simulink model "Task1simu"  (R2020b)
settings: Solver=VariableStepAuto  StartTime=0.0  StopTime=10  RelTol=1e-3
values from neighbouring files (symbols this model uses):
  A = [0,1,0,0;0,0,-m*g/M,0;0,0,0,1;0,0,(M+m)*g/(M*l),0]    [Task1.m]    (also in Task2.m = [-a*m1, a, 0)
  AGC = A-G*c    [Task1.m]
  b = [0;1/M;0;-1/(M*l)]    [Task1.m]    (also in Task2.m = 14.28)
  c = [1,0,0,0]    [Task1.m]    (also in Task2.m = 1)
  G = K2'    [Task1.m]
  K = place(A,b,P1)    [Task1.m]    (also in Task2.m = inv(P)*V)
  KH = K-c    [Task1.m]
  KH1 = K3(1,1:4)    [Task1.m]
  KH2 = -K3(1,5)    [Task1.m]
settings Model: Creator=CLINT  LastModifiedBy=CLINT

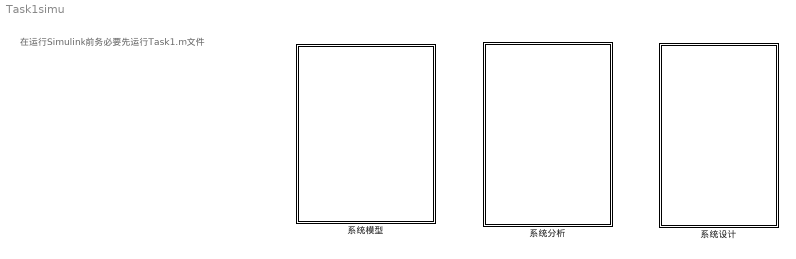
== system Task1simu ==
  note: 在运行Simulink前务必要先运行Task1.m文件
  系统分析 : Subsystem
  系统模型 : Subsystem
  系统设计 : Subsystem

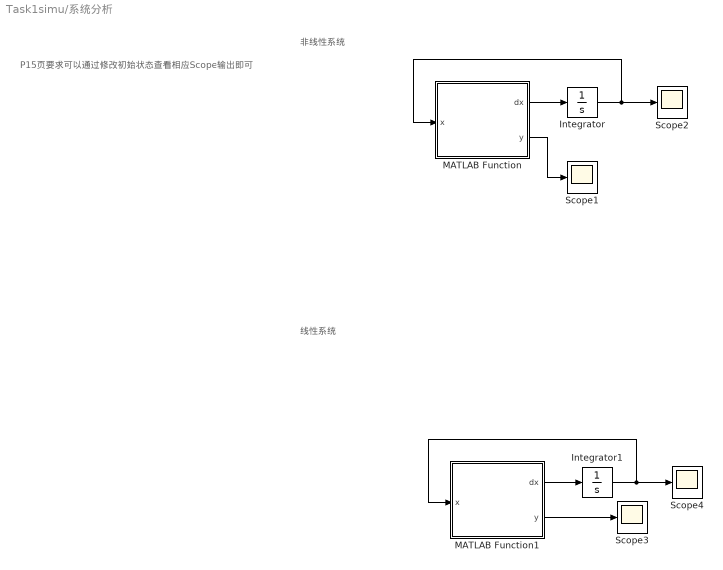
== system Task1simu/系统分析 ==
  note: P15页要求可以通过修改初始状态查看相应Scope输出即可
  note: 非线性系统
  note: 线性系统
  Integrator : Integrator  InitialCondition=[0;0;0.1;0]
  Integrator1 : Integrator  InitialCondition=[0;0;0.1;0]
  MATLAB Function : MATLAB Function  TreatAsAtomicUnit=on
  MATLAB Function1 : MATLAB Function  TreatAsAtomicUnit=on
  Scope{1..4} (4 alike) : Scope
  wires:
  MATLAB Function1/2(y) -> Scope3/1
  Integrator1/1 -> Scope4/1, MATLAB Function1/1(x)
  MATLAB Function/2(y) -> Scope1/1
  MATLAB Function/1(dx) -> Integrator/1
  Integrator/1 -> Scope2/1, MATLAB Function/1(x)
  MATLAB Function1/1(dx) -> Integrator1/1

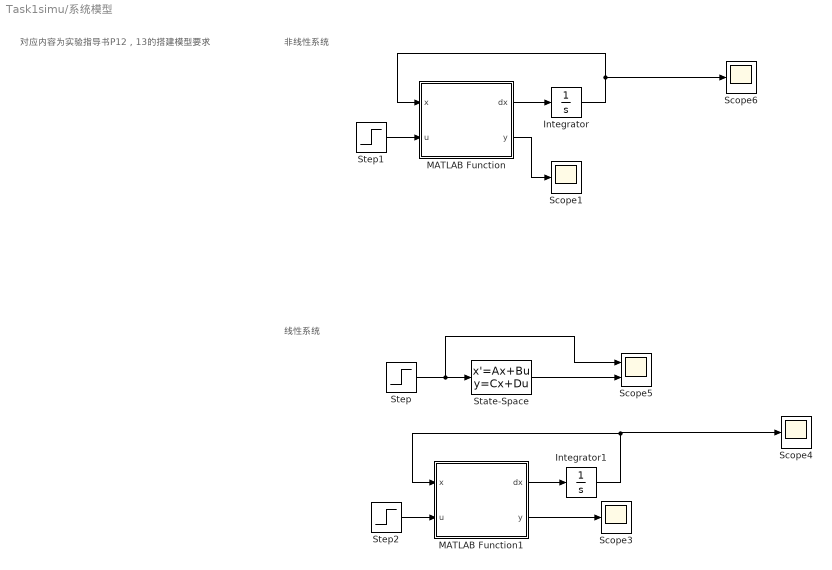
== system Task1simu/系统模型 ==
  note: 非线性系统
  note: 线性系统
  note: 对应内容为实验指导书P12，13的搭建模型要求
  Integrator : Integrator  InitialCondition=[0;0;0;0]
  Integrator1 : Integrator  InitialCondition=[0.1;0;0.1;0]
  MATLAB Function : MATLAB Function  TreatAsAtomicUnit=on
  MATLAB Function1 : MATLAB Function  TreatAsAtomicUnit=on
  Scope{1,3..4,6} (4 alike) : Scope
  Scope5 : Scope  NumInputPorts=2
  State-Space : StateSpace  A=A  B=b  C=c  D=0  InitialCondition=[0;0;0;0]
  Step : Step  SampleTime=0
  Step1 : Step  SampleTime=0
  Step2 : Step  SampleTime=0
  wires:
  MATLAB Function/1(dx) -> Integrator/1
  Step/1 -> Scope5/1, State-Space/1
  MATLAB Function1/1(dx) -> Integrator1/1
  MATLAB Function/2(y) -> Scope1/1
  Integrator1/1 -> Scope4/1, MATLAB Function1/1(x)
  MATLAB Function1/2(y) -> Scope3/1
  Step2/1 -> MATLAB Function1/2(u)
  State-Space/1 -> Scope5/2
  Integrator/1 -> Scope6/1, MATLAB Function/1(x)
  Step1/1 -> MATLAB Function/2(u)

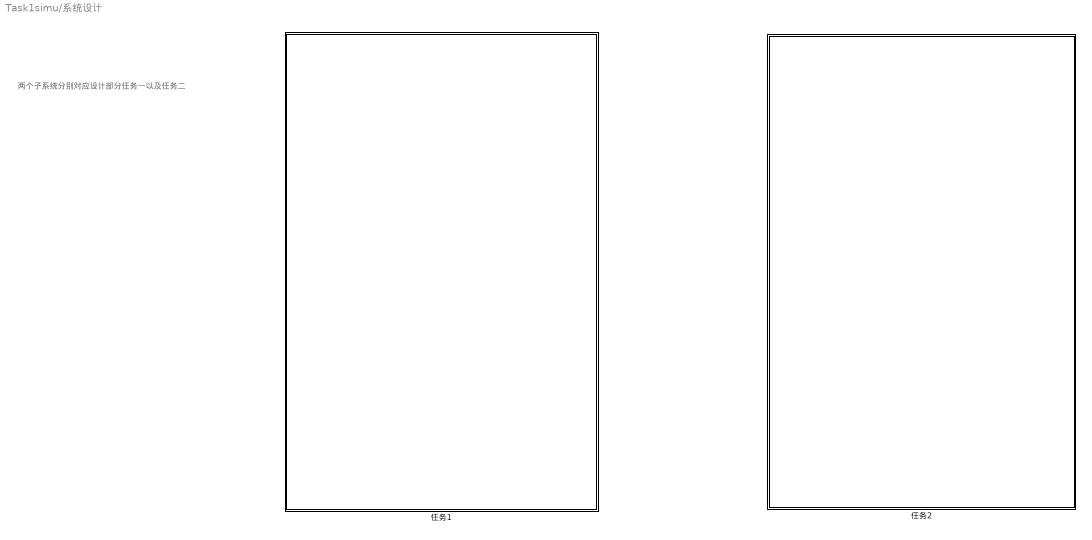
== system Task1simu/系统设计 ==
  note: 两个子系统分别对应设计部分任务一以及任务二
  任务1 : Subsystem
  任务2 : Subsystem

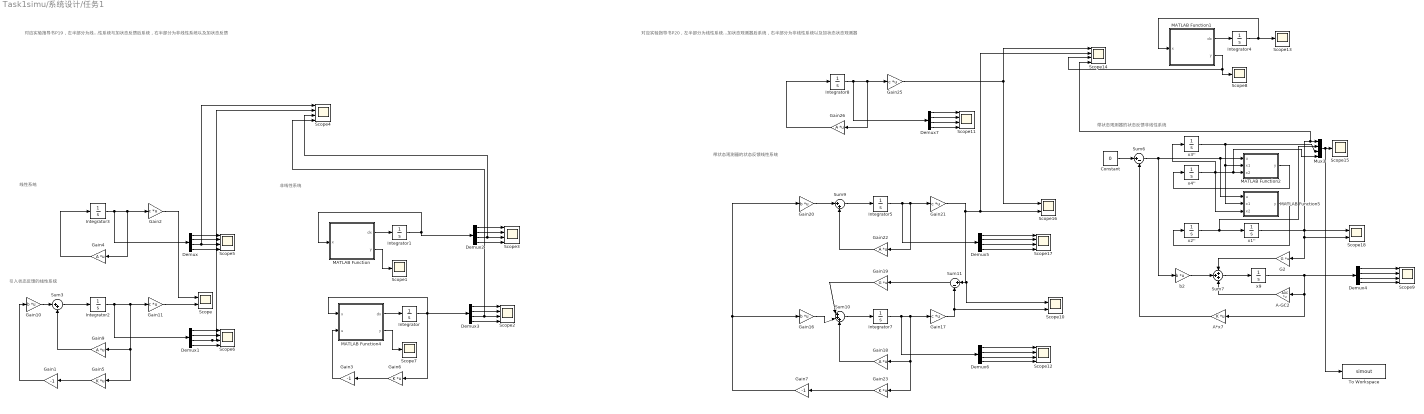
== system Task1simu/系统设计/任务1 ==
  note: 线性系统
  note: 引入状态反馈的线性系统
  note: 非线性系统
  note: 带状态观测器的状态反馈线性系统
  note: 带状态观测器的状态反馈非线性系统
  note: 对应实验指导书P19，左半部分为线性系统与加状态反馈后系统，右半部分为非线性系统以及加状态反馈
  note: 对应实验指导书P20，左半部分为线性系统与加状态观测器后系统，右半部分为非线性系统以及加状态状态观测器
  A*x7 : Gain  Gain=K  Multiplication=Matrix(K*u)
  A-GC2 : Gain  Gain=AGC  Multiplication=Matrix(K*u)
  Constant : Constant  Value=0
  Demux{,1..7} (8 alike) : Demux
  G2 : Gain  Gain=G  Multiplication=Matrix(K*u)
  Gain1 : Gain  Gain=-1
  Gain10 : Gain  Gain=b  Multiplication=Matrix(K*u)
  Gain{2,11,17,21,25} (5 alike) : Gain  Gain=c  Multiplication=Matrix(K*u)
  Gain16 : Gain  Gain=b  Multiplication=Matrix(K*u)
  Gain{4,9,18,22,26} (5 alike) : Gain  Gain=A  Multiplication=Matrix(K*u)
  Gain19 : Gain  Gain=G  Multiplication=Matrix(K*u)
  Gain20 : Gain  Gain=b  Multiplication=Matrix(K*u)
  Gain23 : Gain  Gain=K  Multiplication=Matrix(K*u)
  Gain3 : Gain  Gain=-1
  Gain5 : Gain  Gain=K  Multiplication=Matrix(K*u)
  Gain6 : Gain  Gain=K  Multiplication=Matrix(K*u)
  Gain7 : Gain  Gain=-1
  Integrator{,1..5,8} (7 alike) : Integrator  InitialCondition=[0;0;0.1;0]
  Integrator7 : Integrator  InitialCondition=[0;0.1;0;0.1]
  MATLAB Function : MATLAB Function  TreatAsAtomicUnit=on
  MATLAB Function1 : MATLAB Function  TreatAsAtomicUnit=on
  MATLAB Function2 : MATLAB Function  TreatAsAtomicUnit=on
  MATLAB Function4 : MATLAB Function  TreatAsAtomicUnit=on
  MATLAB Function5 : MATLAB Function  TreatAsAtomicUnit=on
  Mux3 : Mux
  Scope{,10,16,18} (4 alike) : Scope  NumInputPorts=2
  Scope{1,7..8,13,15} (5 alike) : Scope
  Scope{2..6,9,11..12,14,17} (10 alike) : Scope  NumInputPorts=4
  Sum10 : Sum  Inputs=|+++
  Sum11 : Sum  Inputs=|+-
  Sum3 : Sum  Inputs=|++
  Sum6 : Sum  Inputs=|+-
  Sum7 : Sum  Inputs=+++
  Sum9 : Sum  Inputs=|++
  To Workspace : ToWorkspace  VariableName=simout  SaveFormat=Timeseries  SampleTime=-1
  b2 : Gain  Gain=b  Multiplication=Matrix(K*u)
  x1'' : Integrator  InitialCondition=0.1
  x2'' : Integrator  InitialCondition=0.1
  x3'' : Integrator
  "x4'' " : Integrator
  x9 : Integrator  InitialCondition=0.1
  wires:
  Gain4/1 -> Integrator3/1
  Gain11/1 -> Scope/2
  Demux/1 -> Scope5/1
  Integrator2/1 -> Demux1/1, Gain11/1, Gain9/1, Gain5/1
  Integrator/1 -> MATLAB Function4/1(x), Demux3/1, Gain6/1
  Integrator3/1 -> Demux/1, Gain4/1, Gain2/1
  Demux/2 -> Scope5/2
  MATLAB Function/1(dx) -> Integrator1/1
  Demux2/2 -> Scope3/2
  Demux1/4 -> Scope6/4
  Integrator1/1 -> MATLAB Function/1(x), Demux2/1
  MATLAB Function4/2(y) -> Scope7/1
  Demux/3 -> Scope4/1, Scope5/3
  Gain2/1 -> Scope/1
  MATLAB Function/2(y) -> Scope1/1
  Gain5/1 -> Gain1/1
  Sum3/1 -> Integrator2/1
  Gain10/1 -> Sum3/1
  Gain9/1 -> Sum3/2
  Gain1/1 -> Gain10/1
  Demux1/3 -> Scope4/2, Scope6/3
  Demux3/3 -> Scope4/4, Scope2/3
  Demux2/1 -> Scope3/1
  Demux/4 -> Scope5/4
  Gain3/1 -> MATLAB Function4/2(u)
  Demux3/2 -> Scope2/2
  Demux2/3 -> Scope4/3, Scope3/3
  Demux3/4 -> Scope2/4
  Demux2/4 -> Scope3/4
  Demux1/1 -> Scope6/1
  Demux1/2 -> Scope6/2
  Demux3/1 -> Scope2/1
  MATLAB Function4/1(dx) -> Integrator/1
  Gain6/1 -> Gain3/1
  Demux6/2 -> Scope12/2
  Demux4/1 -> Scope9/1
  Gain26/1 -> Integrator8/1
  Gain20/1 -> Sum9/1
  Demux6/3 -> Scope12/3
  x1''/1 -> Scope18/2, G2/1, Scope18/1, Scope14/4, Mux3/1
  Demux4/2 -> Scope9/2
  Demux5/3 -> Scope17/3
  Demux5/1 -> Scope17/1
  Gain16/1 -> Sum10/2
  Demux7/4 -> Scope11/4
  MATLAB Function5/1(y) -> x2''/1
  Integrator7/1 -> Demux6/1, Gain23/1, Gain18/1, Gain17/1
  Demux6/4 -> Scope12/4
  Gain23/1 -> Gain7/1
  Demux7/3 -> Scope11/3
  MATLAB Function2/1(y) -> "x4'' "/1
  Mux3/1 -> To Workspace/1, Scope15/1
  Sum7/1 -> x9/1
  Demux4/3 -> Scope9/3
  Sum9/1 -> Integrator5/1
  Sum11/1 -> Gain19/1
  A*x7/1 -> Sum6/2
  Demux7/2 -> Scope11/2
  x3''/1 -> Mux3/3, MATLAB Function5/2(x1), MATLAB Function2/2(x1)
  "x4'' "/1 -> x3''/1, Mux3/4, MATLAB Function2/3(x2), MATLAB Function5/3(x2)
  Demux4/4 -> Scope9/4
  G2/1 -> Sum7/1
  Demux6/1 -> Scope12/1
  Gain22/1 -> Sum9/2
  b2/1 -> Sum7/2
  Sum10/1 -> Integrator7/1
  Gain19/1 -> Sum10/1
  Integrator5/1 -> Demux5/1, Gain22/1, Gain21/1
  Gain17/1 -> Sum11/2, Scope10/2
  Gain18/1 -> Sum10/3
  x2''/1 -> Mux3/2, x1''/1
  Gain7/1 -> Gain16/1, Gain20/1
  Constant/1 -> Sum6/1
  Gain21/1 -> Scope14/2, Scope16/2, Scope10/1, Sum11/1
  Integrator8/1 -> Demux7/1, Gain26/1, Gain25/1
  Demux7/1 -> Scope11/1
  Integrator4/1 -> Scope13/1, MATLAB Function1/1(x)
  x9/1 -> Demux4/1, A*x7/1, A-GC2/1
  Demux5/2 -> Scope17/2
  Sum6/1 -> MATLAB Function5/1(u), MATLAB Function2/1(u), b2/1
  Gain25/1 -> Scope16/1, Scope14/1
  Demux5/4 -> Scope17/4
  A-GC2/1 -> Sum7/3
  MATLAB Function1/1(dx) -> Integrator4/1
  MATLAB Function1/2(y) -> Scope14/3, Scope8/1

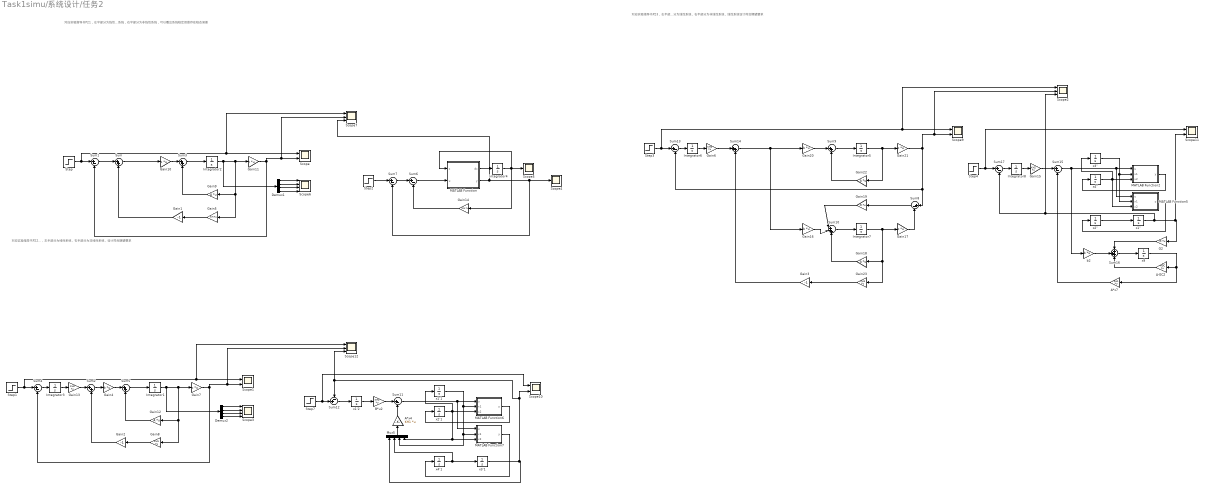
== system Task1simu/系统设计/任务2 ==
  note: 对应实验指导书P21，左半部分为线性系统，右半部分为非线性系统，可以看出系统稳定但是存在稳态误差
  note: 对应实验指导书P22，左半部分为线性系统，右半部分为非线性系统，设计符合期望要求
  note: 对应实验指导书P23，左半部分为线性系统，右半部分为非线性系统，线性系统设计符合期望要求
  A*x4 : Gain  Gain=KH1  Multiplication=Matrix(K*u)
  A*x7 : Gain  Gain=KH1  Multiplication=Matrix(K*u)
  A-GC2 : Gain  Gain=AGC  Multiplication=Matrix(K*u)
  B*u2 : Gain  Gain=KH2  Multiplication=Matrix(K*u)
  Demux1 : Demux
  Demux2 : Demux
  G2 : Gain  Gain=G  Multiplication=Matrix(K*u)
  Gain1 : Gain  Gain=-1
  Gain{4,10,16,20} (4 alike) : Gain  Gain=b  Multiplication=Matrix(K*u)
  Gain{7,11,17,21} (4 alike) : Gain  Gain=c  Multiplication=Matrix(K*u)
  Gain{9,12,18,22} (4 alike) : Gain  Gain=A  Multiplication=Matrix(K*u)
  Gain13 : Gain  Gain=KH2  Multiplication=Matrix(K*u)
  Gain14 : Gain  Gain=KH  Multiplication=Matrix(K*u)
  Gain15 : Gain  Gain=KH2  Multiplication=Matrix(K*u)
  Gain19 : Gain  Gain=G  Multiplication=Matrix(K*u)
  Gain2 : Gain  Gain=-1
  Gain23 : Gain  Gain=KH1  Multiplication=Matrix(K*u)
  Gain3 : Gain  Gain=-1
  Gain5 : Gain  Gain=KH  Multiplication=Matrix(K*u)
  Gain6 : Gain  Gain=KH2  Multiplication=Matrix(K*u)
  Gain8 : Gain  Gain=KH1  Multiplication=Matrix(K*u)
  Integrator1 : Integrator  InitialCondition=[0;0;0;0]
  Integrator2 : Integrator  InitialCondition=[0;0;0;0]
  Integrator3 : Integrator
  Integrator4 : Integrator  InitialCondition=[0;0;0;0]
  Integrator5 : Integrator  InitialCondition=[0;0;0.1;0]
  Integrator6 : Integrator
  Integrator7 : Integrator  InitialCondition=[0;0.1;0;0.1]
  Integrator8 : Integrator
  MATLAB Function : MATLAB Function  TreatAsAtomicUnit=on
  MATLAB Function2 : MATLAB Function  TreatAsAtomicUnit=on
  MATLAB Function5 : MATLAB Function  TreatAsAtomicUnit=on
  MATLAB Function6 : MATLAB Function  TreatAsAtomicUnit=on
  MATLAB Function7 : MATLAB Function  TreatAsAtomicUnit=on
  Mux5 : Mux
  Scope{,1,9..11} (5 alike) : Scope  NumInputPorts=2
  Scope12 : Scope  NumInputPorts=3
  Scope2 : Scope  NumInputPorts=3
  Scope3 : Scope  NumInputPorts=4
  Scope4 : Scope
  Scope5 : Scope
  Scope6 : Scope  NumInputPorts=4
  Scope7 : Scope  NumInputPorts=3
  Step{,1..4,7} (6 alike) : Step  SampleTime=0
  Sum{,2..3,5,9,14} (6 alike) : Sum  Inputs=|++
  Sum{1,4,6..8,11,13,15,17} (9 alike) : Sum  Inputs=|+-
  Sum10 : Sum  Inputs=|+++
  Sum12 : Sum  Inputs=-+|
  Sum16 : Sum  Inputs=+++
  b2 : Gain  Gain=b  Multiplication=Matrix(K*u)
  x1'' : Integrator  InitialCondition=0.1
  x1‘1 : Integrator  InitialCondition=0.1
  x1‘2 : Integrator
  x2'' : Integrator  InitialCondition=0.1
  x2’1 : Integrator  InitialCondition=0.1
  x3'' : Integrator
  x3’1 : Integrator  InitialCondition=0.1
  "x4'' " : Integrator
  x4‘1 : Integrator  InitialCondition=0.1
  x9 : Integrator  InitialCondition=0.1
  wires:
  Gain9/1 -> Sum3/2
  x2’1/1 -> MATLAB Function6/3(x2), x1‘1/1, Mux5/4, MATLAB Function7/3(x2)
  x3’1/1 -> Scope12/3, Sum12/1, Scope10/2, Mux5/1
  "x4'' "/1 -> x3''/1, MATLAB Function2/3(x2), MATLAB Function5/3(x2)
  MATLAB Function2/1(y) -> "x4'' "/1
  Mux5/1 -> A*x4/1
  Demux2/1 -> Scope3/1
  Sum6/1 -> MATLAB Function/2(u)
  Integrator2/1 -> Demux1/1, Gain11/1, Gain9/1, Gain5/1
  MATLAB Function/2(y) -> Scope7/3, Sum7/2, Scope4/1
  Integrator1/1 -> Demux2/1, Gain7/1, Gain12/1, Gain8/1
  x1''/1 -> Scope11/2, G2/1, Scope2/3, Sum17/2
  Step7/1 -> Sum12/2, Scope10/1
  Step2/1 -> Sum7/1
  Gain8/1 -> Gain2/1
  Step/1 -> Scope7/1, Scope/1, Sum1/1
  A*x7/1 -> Sum15/2
  Step1/1 -> Scope12/1, Scope1/1, Sum4/1
  Gain2/1 -> Sum2/2
  Sum9/1 -> Integrator5/1
  Gain7/1 -> Sum4/2, Scope12/2, Scope1/2
  Sum10/1 -> Integrator7/1
  Gain10/1 -> Sum3/1
  Gain5/1 -> Gain1/1
  x4‘1/1 -> Mux5/2, x3’1/1
  Gain13/1 -> Sum2/1
  B*u2/1 -> Sum11/1
  Sum7/1 -> Sum6/1
  A-GC2/1 -> Sum16/3
  Demux1/3 -> Scope6/3
  Sum2/1 -> Gain4/1
  Sum15/1 -> MATLAB Function5/1(u), MATLAB Function2/1(u), b2/1
  x3''/1 -> MATLAB Function5/2(x1), MATLAB Function2/2(x1)
  Gain1/1 -> Sum/2
  Demux1/4 -> Scope6/4
  Sum1/1 -> Sum/1
  Sum/1 -> Gain10/1
  Gain11/1 -> Sum1/2, Scope7/2, Scope/2
  Sum11/1 -> MATLAB Function6/1(u), MATLAB Function7/1(u)
  Sum3/1 -> Integrator2/1
  Integrator4/1 -> Gain14/1, Scope5/1, MATLAB Function/1(x)
  Integrator5/1 -> Gain22/1, Gain21/1
  Demux1/2 -> Scope6/2
  Gain4/1 -> Sum5/1
  Sum13/1 -> Integrator6/1
  Sum5/1 -> Integrator1/1
  Demux1/1 -> Scope6/1
  Integrator3/1 -> Gain13/1
  x1‘1/1 -> Mux5/3, MATLAB Function7/2(x1), MATLAB Function6/2(x1)
  Demux2/3 -> Scope3/3
  Demux2/4 -> Scope3/4
  Gain12/1 -> Sum5/2
  Demux2/2 -> Scope3/2
  Sum4/1 -> Integrator3/1
  MATLAB Function/1(dx) -> Integrator4/1
  Gain14/1 -> Sum6/2
  b2/1 -> Sum16/2
  G2/1 -> Sum16/1
  A*x4/1 -> Sum11/2
  MATLAB Function5/1(y) -> x2''/1
  x2''/1 -> x1''/1
  Sum16/1 -> x9/1
  x9/1 -> A*x7/1, A-GC2/1
  Sum14/1 -> Gain16/1, Gain20/1
  Gain17/1 -> Sum8/2
  Step4/1 -> Scope11/1, Sum17/1
  MATLAB Function6/1(y) -> x2’1/1
  Gain21/1 -> Scope2/2, Scope9/2, Sum13/2, Sum8/1
  Sum12/1 -> x1‘2/1
  x1‘2/1 -> B*u2/1
  MATLAB Function7/1(y) -> x4‘1/1
  Step3/1 -> Scope2/1, Scope9/1, Sum13/1
  Gain6/1 -> Sum14/1
  Gain3/1 -> Sum14/2
  Sum17/1 -> Integrator8/1
  Integrator8/1 -> Gain15/1
  Gain20/1 -> Sum9/1
  Gain18/1 -> Sum10/3
  Gain16/1 -> Sum10/2
  Gain23/1 -> Gain3/1
  Integrator6/1 -> Gain6/1
  Integrator7/1 -> Gain23/1, Gain18/1, Gain17/1
  Gain19/1 -> Sum10/1
  Gain22/1 -> Sum9/2
  Sum8/1 -> Gain19/1
  Gain15/1 -> Sum15/1

== matlab function Task1simu/系统模型/MATLAB Function1 ==
  data: x input; dx output; u input; y output
function [dx,y] = fcn(x,u)
dx = zeros(4,1);
M = 1;
m = 0.1;
l = 0.5;
g = 9.8;
dx(1) = x(2);
dx(2) = -m*g*x(3)/M+u/M;
dx(3) = x(4);
dx(4) = (M+m)*g*x(3)/(M*l)-u/(M*l);
y = x(1);

== matlab function Task1simu/系统设计/任务2/MATLAB Function7 ==
  data: u input; y output; x1 input; x2 input
function y = fcn(u, x1, x2)

y = (u+0.05*sin(x1)*x2*x2-cos(x1)*sin(x1))/(1.1-0.1*cos(x1)*cos(x1));

== matlab function Task1simu/系统设计/任务2/MATLAB Function2 ==
  data: u input; y output; x1 input; x2 input
function y = fcn(u,x1,x2)

y = (u*cos(x1)-11*sin(x1)+0.05*sin(x1)*cos(x1)*x2*x2)/(0.05*cos(x1)*cos(x1)-0.55);

== matlab function Task1simu/系统设计/任务2/MATLAB Function5 ==
  data: u input; y output; x1 input; x2 input
function y = fcn(u,x1,x2)

y = (u+0.05*sin(x1)*x2*x2-cos(x1)*sin(x1))/(1.1-0.1*cos(x1)*cos(x1));

== matlab function Task1simu/系统模型/MATLAB Function ==
  data: x input; dx output; u input; y output
function [dx,y] = fcn(x,u)
dx = zeros(4,1);
M = 1;
m = 0.1;
l = 0.5;
g = 9.8;
dx(1) = x(2);
dx(2) = (u+m*l*x(4)^2*sin(x(3))-m*g*sin(x(3))*cos(x(3)))/(M+m-m*cos(x(3))^2);
dx(3) = x(4);
dx(4) = (-u*cos(x(3))+(M+m)*g*sin(x(3))-m*l*x(4)^2*sin(x(3))*cos(x(3)))/((M+m)*l-m*l*cos(x(3))^2);
y = x(1);

== matlab function Task1simu/系统分析/MATLAB Function ==
  data: x input; dx output; y output
function [dx,y] = fcn(x)
dx = zeros(4,1);
M = 1;
m = 0.1;
l = 0.5;
g = 9.8;
dx(1) = x(2);
dx(2) = (m*l*x(4)^2*sin(x(3))-m*g*sin(x(3))*cos(x(3)))/(M+m-m*cos(x(3))^2);
dx(3) = x(4);
dx(4) = ((M+m)*g*sin(x(3))-m*l*x(4)^2*sin(x(3))*cos(x(3)))/((M+m)*l-m*l*cos(x(3))^2);
y = x(1);

== matlab function Task1simu/系统分析/MATLAB Function1 ==
  data: x input; dx output; y output
function [dx,y] = fcn(x)
dx = zeros(4,1);
M = 1;
m = 0.1;
l = 0.5;
g = 9.8;
dx(1) = x(2);
dx(2) = -m*g*x(3)/M;
dx(3) = x(4);
dx(4) = (M+m)*g*x(3)/(M*l);
y = x(1);

== matlab function Task1simu/系统设计/任务1/MATLAB Function ==
  data: x input; dx output; y output
function [dx,y] = fcn(x)
dx = zeros(4,1);
M = 1;
m = 0.1;
l = 0.5;
g = 9.8;
dx(1) = x(2);
dx(2) = (m*l*x(4)^2*sin(x(3))-m*g*sin(x(3))*cos(x(3)))/(M+m-m*cos(x(3))^2);
dx(3) = x(4);
dx(4) = ((M+m)*g*sin(x(3))-m*l*x(4)^2*sin(x(3))*cos(x(3)))/((M+m)*l-m*l*cos(x(3))^2);
y = x(1);

== matlab function Task1simu/系统设计/任务1/MATLAB Function2 ==
  data: u input; y output; x1 input; x2 input
function y = fcn(u,x1,x2)

y = (u*cos(x1)-11*sin(x1)+0.05*sin(x1)*cos(x1)*x2*x2)/(0.05*cos(x1)*cos(x1)-0.55);

== matlab function Task1simu/系统设计/任务1/MATLAB Function5 ==
  data: u input; y output; x1 input; x2 input
function y = fcn(u,x1,x2)

y = (u+0.05*sin(x1)*x2*x2-cos(x1)*sin(x1))/(1.1-0.1*cos(x1)*cos(x1));

== matlab function Task1simu/系统设计/任务1/MATLAB Function1 ==
  data: x input; dx output; y output
function [dx,y] = fcn(x)
dx = zeros(4,1);
M = 1;
m = 0.1;
l = 0.5;
g = 9.8;
dx(1) = x(2);
dx(2) = (m*l*x(4)^2*sin(x(3))-m*g*sin(x(3))*cos(x(3)))/(M+m-m*cos(x(3))^2);
dx(3) = x(4);
dx(4) = ((M+m)*g*sin(x(3))-m*l*x(4)^2*sin(x(3))*cos(x(3)))/((M+m)*l-m*l*cos(x(3))^2);
y = x(1);

== matlab function Task1simu/系统设计/任务1/MATLAB Function4 ==
  data: x input; dx output; y output; u input
function [dx,y] = fcn(x,u)
dx = zeros(4,1);
M = 1;
m = 0.1;
l = 0.5;
g = 9.8;
dx(1) = x(2);
dx(2) = (u+m*l*x(4)^2*sin(x(3))-m*g*sin(x(3))*cos(x(3)))/(M+m-m*cos(x(3))^2);
dx(3) = x(4);
dx(4) = (-u*cos(x(3))+(M+m)*g*sin(x(3))-m*l*x(4)^2*sin(x(3))*cos(x(3)))/((M+m)*l-m*l*cos(x(3))^2);
y = x(1);

== matlab function Task1simu/系统设计/任务2/MATLAB Function ==
  data: x input; dx output; u input; y output
function [dx,y] = fcn(x,u)
dx = zeros(4,1);
M = 1;
m = 0.1;
l = 0.5;
g = 9.8;
dx(1) = x(2);
dx(2) = (u+m*l*x(4)^2*sin(x(3))-m*g*sin(x(3))*cos(x(3)))/(M+m-m*cos(x(3))^2);
dx(3) = x(4);
dx(4) = (-u*cos(x(3))+(M+m)*g*sin(x(3))-m*l*x(4)^2*sin(x(3))*cos(x(3)))/((M+m)*l-m*l*cos(x(3))^2);
y = x(1);

== matlab function Task1simu/系统设计/任务2/MATLAB Function6 ==
  data: u input; y output; x1 input; x2 input
function y = fcn(u, x1, x2)

y = (u*cos(x1)-11*sin(x1)+0.05*sin(x1)*cos(x1)*x2*x2)/(0.05*cos(x1)*cos(x1)-0.55);
